simulink model "three_phase"  (R2025b)
settings: Solver=VariableStepAuto  StartTime=0.0  StopTime=5/60  RelTol=1e-3
InitFcn:
  | Ts = 5e-5;
undefined symbols (not defined in the file or in its folder): Ran, Rbn, Rcn
libraries: nesl_utility x24, fl_lib x21, ee_lib x3, eePowerMeasurement x3
settings Model: Creator=gdudgeon  LastModifiedBy=gdudgeon
settings DataIOCC: SaveOutput=off  SignalLogging=off  DSMLogging=off  InspectSignalLogs=on  SaveTime=off  ReturnWorkspaceOutputs=off
settings OptimizationCC: ReuseModelBlockBuffer=off
settings DebuggingCC: UnconnectedInputMsg=warning  UnconnectedOutputMsg=warning  UnconnectedLineMsg=warning
settings ModelReferenceCC: EnableRefExpFcnMdlSchedulingChecks=on
settings RTWCC: GPUComputeCapability=3.5  DLArmComputeVersion=19.05

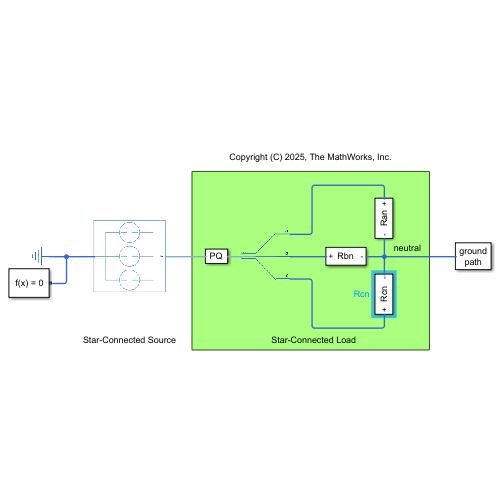
[thumbnail: Simulink's stored preview of the top-level diagram]
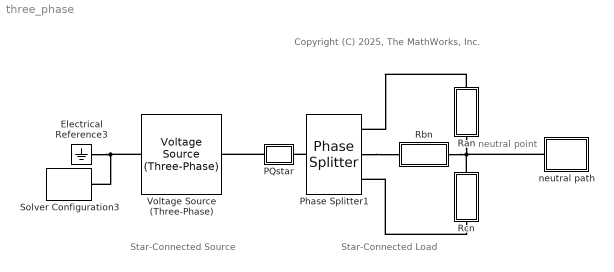
== system three_phase ==
  note: Copyright (C) 2025, The MathWorks, Inc.
  note: Star-Connected Source
  note: neutral point
  note: Star-Connected Load
  Electrical Reference3 : fl_lib/Electrical/Electrical Elements/Electrical Reference
  PQstar : Subsystem
      mask Display: disp('PQ')
  Phase Splitter1 : ee_lib/Connectors & References/Phase Splitter
  Ran : Subsystem
      mask Display: disp('Ran')
  Rbn : Subsystem
      mask Display: disp('Rbn')
  Rcn : Subsystem
      mask Display: disp('Rcn')
  Solver Configuration3 : nesl_utility/Solver Configuration  PhysicalDomain=network_engine_domain  SubClassName=solver  LeftPortType=input  RightPortType=generic  Tones=[]  Harmonics=[]  SimulateNoise=off  Profile=off  UseLocalSampling=off  EnableSwitchedLinearOptims=on  FrequencyDomain=off  UseCCode=off  RelTol=0.001  AbsTol=1e-06  MinStep=1e-09  ToWorkspace=off  RevertToSquareIcSolve=off  NumHomotopyIterations=100  PhasorMode=off  PhasorModeNumHarmonics=1  ConsistencySolver=NEWTON_FTOL  IndexReductionMethod=DerivativeReplacement  DoDC=off  ResidualTolerance=1e-09  ConsistencyTolSource=GLOBAL  ConsistencyAbsTol=0.001  ConsistencyRelTol=0.001  ConsistencyTolFactor=0.001  UseLocalSolver=on  LocalSolverChoice=NE_TRAPEZOIDAL_ADVANCER  ResolveIndetEquations=on  FunctionEvalNumThread=1  LocalSolverSampleTime=Ts  DoFixedCost=on  MaxNonlinIter=3  MaxModeIter=2  ComputeImpulses=off  ImpulseIterations=2  LinearAlgebra=auto  LinearAlgebraNumThread=0  EquationFormulation=NE_TIME_EF  DelaysMemoryBudget=1024  AutomaticFiltering=on  FilteringTimeConstant=0.001  PartitionStorageMethod=AS_NEEDED  PartitionMemoryBudget=1024  PartitionMethod=ROBUST  MultibodyUseLocalSolver=off  MultibodyLocalSolverChoice=ODE1  MultibodyLocalSolverSampleTime=0.001
  Voltage Source (Three-Phase) : ee_lib/Sources/Voltage Source (Three-Phase)  vline_rms=sqrt(3) * 1 / sqrt(2) V  shift=0 deg  freq=60 Hz  impedance_option=0  SShortCircuit=1e6 A*V  XR=15  R=0.01 Ohm  L=3.97e-4 H  harmonic_option=0  harmonic_orders=[5, 7, 11, 13]  harmonic_ratios=[.1, .1, .1, .1]  G_parasitic=0 1/Ohm  I_specify=off  I_priority=None  I=[0, 0, 0] A  I_nominal_specify=off  I_nominal_value=1  I_nominal_unit=A
  neutral path : Subsystem
      mask Display: disp('ground\npath')
  connections:
  Electrical Reference3/LConn1 -- Voltage Source (Three-Phase)/LConn1 -- Solver Configuration3/RConn1
  Rbn/RConn1 -- Rcn/RConn1 -- neutral path/LConn1 -- Ran/RConn1
  Ran/LConn1 -- Phase Splitter1/RConn1
  Phase Splitter1/RConn2 -- Rbn/LConn1
  Rcn/LConn1 -- Phase Splitter1/RConn3
  PQstar/LConn1 -- Voltage Source (Three-Phase)/RConn1
  Phase Splitter1/LConn1 -- PQstar/RConn1

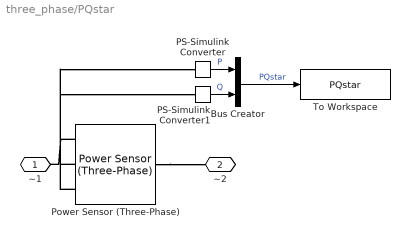
== system three_phase/PQstar ==
  Bus Creator : BusCreator  Inputs=2
  PS-Simulink Converter : nesl_utility/PS-Simulink Converter  PhysicalDomain=network_engine_domain  SubClassName=ps_output  LeftPortType=input  RightPortType=output  PseudoPeriodic=off  Frequencies=[]  VectorFormat=1-D array  Unit=W  AffineConversion=off
  PS-Simulink Converter1 : nesl_utility/PS-Simulink Converter  PhysicalDomain=network_engine_domain  SubClassName=ps_output  LeftPortType=input  RightPortType=output  PseudoPeriodic=off  Frequencies=[]  VectorFormat=1-D array  Unit=V*A  AffineConversion=off
  Power Sensor (Three-Phase) : ee_lib/Sensors & Transducers/Power Sensor (Three-Phase)  load_type=ee.enum.passive.type_balanced.balanced  f0=60 Hz
      settings: InternalSimscapePortConfiguration="{\"Bottom\":[],\"Left\":[{\"id\":\"N1\",\"label\":\"~1\",\"type\":\"foundation.electrical.three_phase\"}],\"Right\":[{\"id\":\"N2\",\"label\":\"~2\",\"type\":\"foundation.electrical.three_phase\"}],\"Top\":[{\"id\":\"Pm\",\"label\":\"P\",\"type\":\"output\"},{\"id\":\"Qm\",\"label\":\"Q\",\"type\":\"output\"}]}"
  To Workspace : ToWorkspace  VariableName=PQstar  SaveFormat=Timeseries  SampleTime=-1
  ~1 : PMIOPort  Side=Left
  ~2 : PMIOPort  Port=2  Side=Right
  wires:
  PS-Simulink Converter/1 -> Bus Creator/1  "P"
  PS-Simulink Converter1/1 -> Bus Creator/2  "Q"
  Bus Creator/1 -> To Workspace/1  "PQstar"
  connections:
  Power Sensor (Three-Phase)/RConn1 -- ~2/RConn1
  Power Sensor (Three-Phase)/LConn1 -- ~1/RConn1
  Power Sensor (Three-Phase)/LConn2 -- PS-Simulink Converter/LConn1
  Power Sensor (Three-Phase)/LConn3 -- PS-Simulink Converter1/LConn1

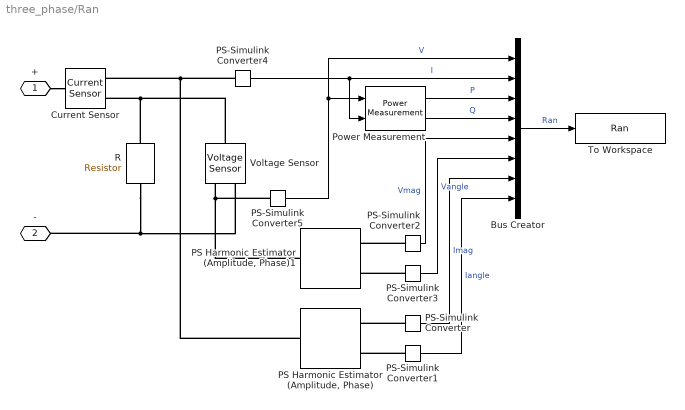
== system three_phase/Ran ==
  Bus Creator : BusCreator  Inputs=8
  Current Sensor : fl_lib/Electrical/Electrical Sensors/Current Sensor
  "PS Harmonic Estimator (Amplitude, Phase)" : fl_lib/Physical Signals/Periodic Operators/PS Harmonic Estimator (Amplitude, Phase)  f0=60 Hz  n=1  amplMin=0.001 A
      settings: InternalSimscapePortConfiguration="{\"Bottom\":[],\"Left\":[{\"id\":\"I\",\"label\":\"I\",\"type\":\"input\"}],\"Right\":[{\"id\":\"A\",\"label\":\"A\",\"type\":\"output\"},{\"id\":\"Phi\",\"label\":\"Phi\",\"type\":\"output\"}],\"Top\":[]}"
  "PS Harmonic Estimator (Amplitude, Phase)1" : fl_lib/Physical Signals/Periodic Operators/PS Harmonic Estimator (Amplitude, Phase)  f0=60 Hz  n=1  amplMin=0.001 V
      settings: InternalSimscapePortConfiguration="{\"Bottom\":[],\"Left\":[{\"id\":\"I\",\"label\":\"I\",\"type\":\"input\"}],\"Right\":[{\"id\":\"A\",\"label\":\"A\",\"type\":\"output\"},{\"id\":\"Phi\",\"label\":\"Phi\",\"type\":\"output\"}],\"Top\":[]}"
  PS-Simulink Converter{,1..5} (6 alike) : nesl_utility/PS-Simulink Converter  PhysicalDomain=network_engine_domain  SubClassName=ps_output  LeftPortType=input  RightPortType=output  PseudoPeriodic=off  Frequencies=[]  VectorFormat=1-D array  Unit=inherit  AffineConversion=off
  Power Measurement : eePowerMeasurement/Power Measurement  LabelModeActiveChoice=Discrete  F=60  K=1  Ts=Ts
  R : fl_lib/Electrical/Electrical Elements/Resistor  R=Ran Ohm  i_specify=off  i_priority=None  i=0 A  i_nominal_specify=off  i_nominal_value=1  i_nominal_unit=A  v_specify=off  v_priority=None  v=0 V  v_nominal_specify=off  v_nominal_value=1  v_nominal_unit=V
  To Workspace : ToWorkspace  VariableName=Ran  SaveFormat=Timeseries  SampleTime=-1
  Voltage Sensor : fl_lib/Electrical/Electrical Sensors/Voltage Sensor
  + : PMIOPort  Side=Left
  - : PMIOPort  Port=2  Side=Right
  wires:
  Bus Creator/1 -> To Workspace/1  "Ran"
  PS-Simulink Converter1/1 -> Bus Creator/8  "Iangle"
  PS-Simulink Converter/1 -> Bus Creator/7  "Imag"
  PS-Simulink Converter3/1 -> Bus Creator/6  "Vangle"
  PS-Simulink Converter2/1 -> Bus Creator/5  "Vmag"
  Power Measurement/1 -> Bus Creator/3  "P"
  Power Measurement/2 -> Bus Creator/4  "Q"
  PS-Simulink Converter4/1 -> Power Measurement/2, Bus Creator/2  "I"
  PS-Simulink Converter5/1 -> Power Measurement/1, Bus Creator/1  "V"
  connections:
  +/RConn1 -- Current Sensor/LConn1
  Voltage Sensor/LConn1 -- R/LConn1 -- Current Sensor/RConn2
  PS-Simulink Converter3/LConn1 -- "PS Harmonic Estimator (Amplitude, Phase)1"/RConn2
  PS-Simulink Converter2/LConn1 -- "PS Harmonic Estimator (Amplitude, Phase)1"/RConn1
  PS-Simulink Converter1/LConn1 -- "PS Harmonic Estimator (Amplitude, Phase)"/RConn2
  PS-Simulink Converter/LConn1 -- "PS Harmonic Estimator (Amplitude, Phase)"/RConn1
  PS-Simulink Converter5/LConn1 -- "PS Harmonic Estimator (Amplitude, Phase)1"/LConn1 -- Voltage Sensor/RConn1
  Current Sensor/RConn1 -- "PS Harmonic Estimator (Amplitude, Phase)"/LConn1 -- PS-Simulink Converter4/LConn1
  Voltage Sensor/RConn2 -- -/RConn1 -- R/RConn1

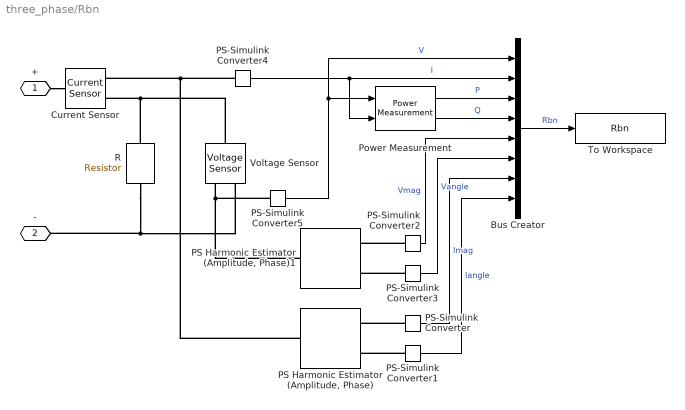
== system three_phase/Rbn ==
  Bus Creator : BusCreator  Inputs=8
  Current Sensor : fl_lib/Electrical/Electrical Sensors/Current Sensor
  "PS Harmonic Estimator (Amplitude, Phase)" : fl_lib/Physical Signals/Periodic Operators/PS Harmonic Estimator (Amplitude, Phase)  f0=60 Hz  n=1  amplMin=0.001 A
      settings: InternalSimscapePortConfiguration="{\"Bottom\":[],\"Left\":[{\"id\":\"I\",\"label\":\"I\",\"type\":\"input\"}],\"Right\":[{\"id\":\"A\",\"label\":\"A\",\"type\":\"output\"},{\"id\":\"Phi\",\"label\":\"Phi\",\"type\":\"output\"}],\"Top\":[]}"
  "PS Harmonic Estimator (Amplitude, Phase)1" : fl_lib/Physical Signals/Periodic Operators/PS Harmonic Estimator (Amplitude, Phase)  f0=60 Hz  n=1  amplMin=0.001 V
      settings: InternalSimscapePortConfiguration="{\"Bottom\":[],\"Left\":[{\"id\":\"I\",\"label\":\"I\",\"type\":\"input\"}],\"Right\":[{\"id\":\"A\",\"label\":\"A\",\"type\":\"output\"},{\"id\":\"Phi\",\"label\":\"Phi\",\"type\":\"output\"}],\"Top\":[]}"
  PS-Simulink Converter{,1..5} (6 alike) : nesl_utility/PS-Simulink Converter  PhysicalDomain=network_engine_domain  SubClassName=ps_output  LeftPortType=input  RightPortType=output  PseudoPeriodic=off  Frequencies=[]  VectorFormat=1-D array  Unit=inherit  AffineConversion=off
  Power Measurement : eePowerMeasurement/Power Measurement  LabelModeActiveChoice=Discrete  F=60  K=1  Ts=Ts
  R : fl_lib/Electrical/Electrical Elements/Resistor  R=Rbn Ohm  i_specify=off  i_priority=None  i=0 A  i_nominal_specify=off  i_nominal_value=1  i_nominal_unit=A  v_specify=off  v_priority=None  v=0 V  v_nominal_specify=off  v_nominal_value=1  v_nominal_unit=V
  To Workspace : ToWorkspace  VariableName=Rbn  SaveFormat=Timeseries  SampleTime=-1
  Voltage Sensor : fl_lib/Electrical/Electrical Sensors/Voltage Sensor
  + : PMIOPort  Side=Left
  - : PMIOPort  Port=2  Side=Right
  wires:
  PS-Simulink Converter5/1 -> Power Measurement/1, Bus Creator/1  "V"
  PS-Simulink Converter4/1 -> Power Measurement/2, Bus Creator/2  "I"
  Power Measurement/2 -> Bus Creator/4  "Q"
  Power Measurement/1 -> Bus Creator/3  "P"
  PS-Simulink Converter2/1 -> Bus Creator/5  "Vmag"
  PS-Simulink Converter3/1 -> Bus Creator/6  "Vangle"
  PS-Simulink Converter/1 -> Bus Creator/7  "Imag"
  PS-Simulink Converter1/1 -> Bus Creator/8  "Iangle"
  Bus Creator/1 -> To Workspace/1  "Rbn"
  connections:
  -/RConn1 -- R/RConn1 -- Voltage Sensor/RConn2
  PS-Simulink Converter4/LConn1 -- "PS Harmonic Estimator (Amplitude, Phase)"/LConn1 -- Current Sensor/RConn1
  Voltage Sensor/RConn1 -- "PS Harmonic Estimator (Amplitude, Phase)1"/LConn1 -- PS-Simulink Converter5/LConn1
  PS-Simulink Converter/LConn1 -- "PS Harmonic Estimator (Amplitude, Phase)"/RConn1
  PS-Simulink Converter1/LConn1 -- "PS Harmonic Estimator (Amplitude, Phase)"/RConn2
  PS-Simulink Converter2/LConn1 -- "PS Harmonic Estimator (Amplitude, Phase)1"/RConn1
  PS-Simulink Converter3/LConn1 -- "PS Harmonic Estimator (Amplitude, Phase)1"/RConn2
  R/LConn1 -- Voltage Sensor/LConn1 -- Current Sensor/RConn2
  +/RConn1 -- Current Sensor/LConn1

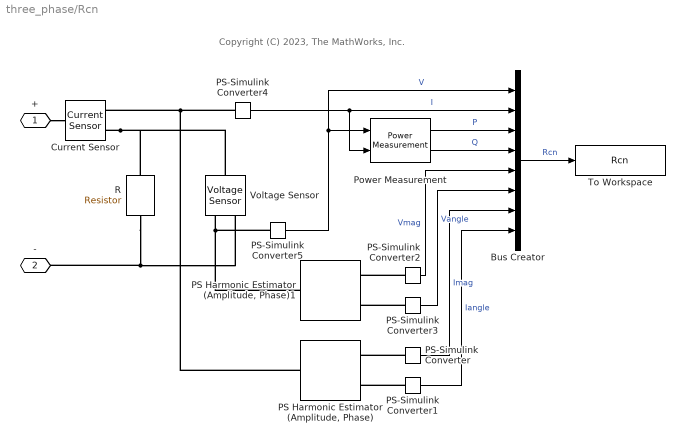
== system three_phase/Rcn ==
  note: Copyright (C) 2023, The MathWorks, Inc.
  Bus Creator : BusCreator  Inputs=8
  Current Sensor : fl_lib/Electrical/Electrical Sensors/Current Sensor
  "PS Harmonic Estimator (Amplitude, Phase)" : fl_lib/Physical Signals/Periodic Operators/PS Harmonic Estimator (Amplitude, Phase)  f0=60 Hz  n=1  amplMin=0.001 A
      settings: InternalSimscapePortConfiguration="{\"Bottom\":[],\"Left\":[{\"id\":\"I\",\"label\":\"I\",\"type\":\"input\"}],\"Right\":[{\"id\":\"A\",\"label\":\"A\",\"type\":\"output\"},{\"id\":\"Phi\",\"label\":\"Phi\",\"type\":\"output\"}],\"Top\":[]}"
  "PS Harmonic Estimator (Amplitude, Phase)1" : fl_lib/Physical Signals/Periodic Operators/PS Harmonic Estimator (Amplitude, Phase)  f0=60 Hz  n=1  amplMin=0.001 V
      settings: InternalSimscapePortConfiguration="{\"Bottom\":[],\"Left\":[{\"id\":\"I\",\"label\":\"I\",\"type\":\"input\"}],\"Right\":[{\"id\":\"A\",\"label\":\"A\",\"type\":\"output\"},{\"id\":\"Phi\",\"label\":\"Phi\",\"type\":\"output\"}],\"Top\":[]}"
  PS-Simulink Converter{,1..5} (6 alike) : nesl_utility/PS-Simulink Converter  PhysicalDomain=network_engine_domain  SubClassName=ps_output  LeftPortType=input  RightPortType=output  PseudoPeriodic=off  Frequencies=[]  VectorFormat=1-D array  Unit=inherit  AffineConversion=off
  Power Measurement : eePowerMeasurement/Power Measurement  LabelModeActiveChoice=Discrete  F=60  K=1  Ts=Ts
  R : fl_lib/Electrical/Electrical Elements/Resistor  R=Rcn Ohm  i_specify=off  i_priority=None  i=0 A  i_nominal_specify=off  i_nominal_value=1  i_nominal_unit=A  v_specify=off  v_priority=None  v=0 V  v_nominal_specify=off  v_nominal_value=1  v_nominal_unit=V
  To Workspace : ToWorkspace  VariableName=Rcn  SaveFormat=Timeseries  SampleTime=-1
  Voltage Sensor : fl_lib/Electrical/Electrical Sensors/Voltage Sensor
  + : PMIOPort  Side=Left
  - : PMIOPort  Port=2  Side=Right
  wires:
  PS-Simulink Converter5/1 -> Power Measurement/1, Bus Creator/1  "V"
  PS-Simulink Converter4/1 -> Power Measurement/2, Bus Creator/2  "I"
  Power Measurement/2 -> Bus Creator/4  "Q"
  Power Measurement/1 -> Bus Creator/3  "P"
  PS-Simulink Converter2/1 -> Bus Creator/5  "Vmag"
  PS-Simulink Converter3/1 -> Bus Creator/6  "Vangle"
  PS-Simulink Converter/1 -> Bus Creator/7  "Imag"
  PS-Simulink Converter1/1 -> Bus Creator/8  "Iangle"
  Bus Creator/1 -> To Workspace/1  "Rcn"
  connections:
  R/RConn1 -- -/RConn1 -- Voltage Sensor/RConn2
  PS-Simulink Converter4/LConn1 -- "PS Harmonic Estimator (Amplitude, Phase)"/LConn1 -- Current Sensor/RConn1
  Voltage Sensor/RConn1 -- "PS Harmonic Estimator (Amplitude, Phase)1"/LConn1 -- PS-Simulink Converter5/LConn1
  PS-Simulink Converter/LConn1 -- "PS Harmonic Estimator (Amplitude, Phase)"/RConn1
  PS-Simulink Converter1/LConn1 -- "PS Harmonic Estimator (Amplitude, Phase)"/RConn2
  PS-Simulink Converter2/LConn1 -- "PS Harmonic Estimator (Amplitude, Phase)1"/RConn1
  PS-Simulink Converter3/LConn1 -- "PS Harmonic Estimator (Amplitude, Phase)1"/RConn2
  Current Sensor/RConn2 -- R/LConn1 -- Voltage Sensor/LConn1
  +/RConn1 -- Current Sensor/LConn1

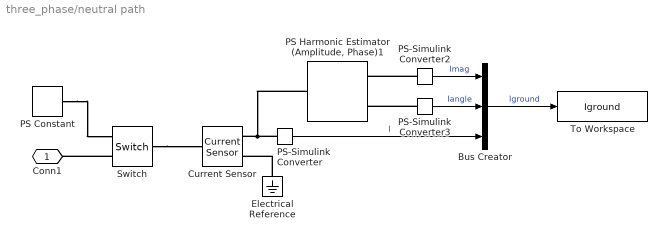
== system three_phase/neutral path ==
  Bus Creator : BusCreator  Inputs=3
  Current Sensor : fl_lib/Electrical/Electrical Sensors/Current Sensor
  Electrical Reference : fl_lib/Electrical/Electrical Elements/Electrical Reference
  PS Constant : fl_lib/Physical Signals/Sources/PS Constant  constant=neutral_path
  "PS Harmonic Estimator (Amplitude, Phase)1" : fl_lib/Physical Signals/Periodic Operators/PS Harmonic Estimator (Amplitude, Phase)  f0=60 Hz  n=1  amplMin=0.001 A
      settings: InternalSimscapePortConfiguration="{\"Bottom\":[],\"Left\":[{\"id\":\"I\",\"label\":\"I\",\"type\":\"input\"}],\"Right\":[{\"id\":\"A\",\"label\":\"A\",\"type\":\"output\"},{\"id\":\"Phi\",\"label\":\"Phi\",\"type\":\"output\"}],\"Top\":[]}"
  PS-Simulink Converter : nesl_utility/PS-Simulink Converter  PhysicalDomain=network_engine_domain  SubClassName=ps_output  LeftPortType=input  RightPortType=output  PseudoPeriodic=off  Frequencies=[]  VectorFormat=1-D array  Unit=inherit  AffineConversion=off
  PS-Simulink Converter2 : nesl_utility/PS-Simulink Converter  PhysicalDomain=network_engine_domain  SubClassName=ps_output  LeftPortType=input  RightPortType=output  PseudoPeriodic=off  Frequencies=[]  VectorFormat=1-D array  Unit=inherit  AffineConversion=off
  PS-Simulink Converter3 : nesl_utility/PS-Simulink Converter  PhysicalDomain=network_engine_domain  SubClassName=ps_output  LeftPortType=input  RightPortType=output  PseudoPeriodic=off  Frequencies=[]  VectorFormat=1-D array  Unit=inherit  AffineConversion=off
  Switch : fl_lib/Electrical/Electrical Elements/Switch  R_closed=0.01 Ohm  G_open=1e-8 1/Ohm  Threshold=0.5  i_specify=off  i_priority=None  i=0 A  i_nominal_specify=off  i_nominal_value=1  i_nominal_unit=A  v_specify=off  v_priority=None  v=0 V  v_nominal_specify=off  v_nominal_value=1  v_nominal_unit=V
  To Workspace : ToWorkspace  VariableName=Iground  SaveFormat=Timeseries  SampleTime=-1
  Conn1 : PMIOPort  Side=Left
  wires:
  Bus Creator/1 -> To Workspace/1  "Iground"
  PS-Simulink Converter2/1 -> Bus Creator/1  "Imag"
  PS-Simulink Converter3/1 -> Bus Creator/2  "Iangle"
  PS-Simulink Converter/1 -> Bus Creator/3  "I"
  connections:
  PS-Simulink Converter/LConn1 -- "PS Harmonic Estimator (Amplitude, Phase)1"/LConn1 -- Current Sensor/RConn1
  Electrical Reference/LConn1 -- Current Sensor/RConn2
  PS-Simulink Converter3/LConn1 -- "PS Harmonic Estimator (Amplitude, Phase)1"/RConn2
  PS-Simulink Converter2/LConn1 -- "PS Harmonic Estimator (Amplitude, Phase)1"/RConn1
  Switch/RConn2 -- Conn1/RConn1
  Switch/LConn1 -- Current Sensor/LConn1
  PS Constant/RConn1 -- Switch/RConn1
